simulink model "BLDC_fuzzy_sim"  (R2017a)
settings: Solver=VariableStepAuto  StartTime=0.0  StopTime=10.0  RelTol=1e-3
values from neighbouring files (symbols this model uses):
  A = [-R/L -Kb/L; Km/J -Kf/J]    [BLDC_par.m]
  B = [1/L; 0]    [BLDC_par.m]
  C = [0 1]    [BLDC_par.m]
  D = [0]    [BLDC_par.m]
libraries: fuzblock x1
settings Model: Creator=Yenchun  LastModifiedBy=Yenchun

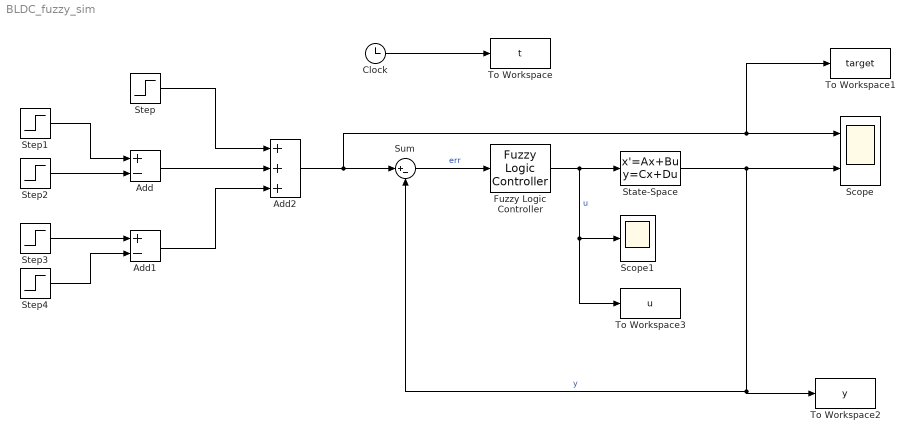
== system BLDC_fuzzy_sim ==
  Add : Sum  Inputs=+-
  Add1 : Sum  Inputs=+-
  Add2 : Sum  Inputs=+++
  Clock : Clock
  Fuzzy Logic Controller : fuzblock/Fuzzy Logic  Controller  fis=readfis('BLDC_fuzzy_controller.fis')
  Scope : Scope  NumInputPorts=2
  Scope1 : Scope
  State-Space : StateSpace  A=A  B=B  C=C  D=D  X0=0
  Step : Step  SampleTime=0
  Step1 : Step  SampleTime=0
  Step2 : Step  SampleTime=0
  Step3 : Step  Before=1  After=0  SampleTime=0
  Step4 : Step  Before=1  After=0  SampleTime=0
  Sum : Sum  Inputs=|+-
  To Workspace : ToWorkspace  VariableName=t  SaveFormat=Timeseries  SampleTime=-1
  To Workspace1 : ToWorkspace  VariableName=target  SaveFormat=Timeseries  SampleTime=-1
  To Workspace2 : ToWorkspace  VariableName=y  SaveFormat=Timeseries  SampleTime=-1
  To Workspace3 : ToWorkspace  VariableName=u  SaveFormat=Timeseries  SampleTime=-1
  wires:
  Add/1 -> Add2/2
  Add1/1 -> Add2/3
  Step1/1 -> Add/1
  Step2/1 -> Add/2
  Step3/1 -> Add1/1
  Step4/1 -> Add1/2
  Step/1 -> Add2/1
  Add2/1 -> To Workspace1/1, Scope/1, Sum/1
  Sum/1 -> Fuzzy Logic Controller/1  "err"
  Fuzzy Logic Controller/1 -> Scope1/1, To Workspace3/1, State-Space/1  "u"
  State-Space/1 -> Sum/2, To Workspace2/1, Scope/2  "y"
  Clock/1 -> To Workspace/1
